simulink model "SIL_PIL_position_controller_model"  (R2023b)
settings: Solver=FixedStepAuto  StartTime=0.0  StopTime=10.0  RelTol=1e-3  EnableMultiTasking=on
undefined symbols (not defined in the file): DiscIntNeverNeededParam, K
settings Model: ExtModeTrigDuration=10  Creator=paoli  LastModifiedBy=paoli
settings OptimizationCC: EnhancedBackFolding=on  PassReuseOutputArgsAs=Individual arguments  ZeroExternalMemoryAtStartup=off  ZeroInternalMemoryAtStartup=off  MaxStackSize=64  OptimizeBlockOrder=speed  DifferentSizesBufferReuse=on  OptimizationCustomize=off  EfficientTunableParamExpr=on
settings DebuggingCC: ParameterTunabilityLossMsg=error
settings HardwareCC: ProdBitPerPointer=32  ProdBitPerSizeT=32  ProdBitPerPtrDiffT=32  ProdLargestAtomicInteger=Long  ProdLargestAtomicFloat=Double  ProdWordSize=32  ProdLongLongMode=on  ProdHWDeviceType=ARM Compatible->ARM Cortex
settings SFSimCC: MATLABDynamicMemAlloc=off
settings RTWCC: Description=Embedded Coder  SystemTargetFile=ert.tlc  HardwareBoard=STM32 Nucleo F401RE  TemplateMakefile=ert_default_tmf  Toolchain=GNU Tools for ARM Embedded Processors  PortableWordSizes=on
settings CodeAppCC: ForceParamTrailComments=on  IgnoreCustomStorageClasses=off  OperatorAnnotations=on  SimulinkDataObjDesc=on  SFDataObjDesc=on  InsertBlockDesc=on
settings ERTTargetCC: ExtModeTransport=3  ExtModeStaticAlloc=on  ExtModeStaticAllocSize=2000  ExtModeMexFile=ext_xcp  ExtModeIntrfLevel=Level2 - Open

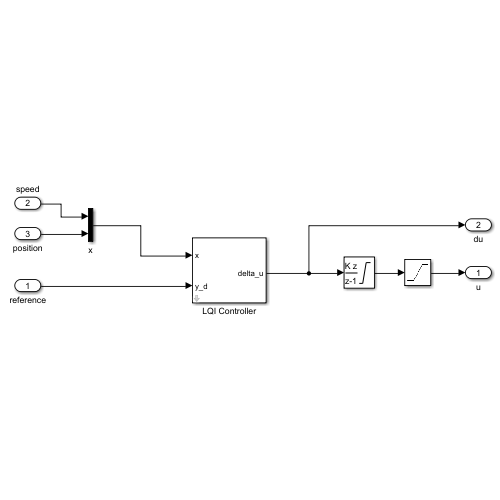
[thumbnail: Simulink's stored preview of the top-level diagram]
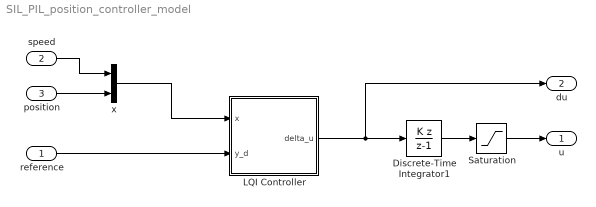
== system SIL_PIL_position_controller_model ==
  reference : Inport
  speed : Inport  Port=2
  position : Inport  Port=3
  Discrete-Time Integrator1 : DiscreteIntegrator  IntegratorMethod=Accumulation: Backward Euler  SampleTime=-1  LimitOutput=on  UpperSaturationLimit=12  LowerSaturationLimit=-12  ICPrevOutput=DiscIntNeverNeededParam  ICPrevScaledInput=DiscIntNeverNeededParam
  LQI Controller : Subsystem  mask{Ts=0.005}
  Saturation : Saturate  UpperLimit=12  LowerLimit=-12
  x : Mux  Inputs=2
  u : Outport
  du : Outport  Port=2
  wires:
  Discrete-Time Integrator1/1 -> Saturation/1
  LQI Controller/1(delta_u) -> du/1, Discrete-Time Integrator1/1
  Saturation/1 -> u/1
  reference/1 -> LQI Controller/2(y_d)
  speed/1 -> x/1
  position/1 -> x/2
  x/1 -> LQI Controller/1(x)

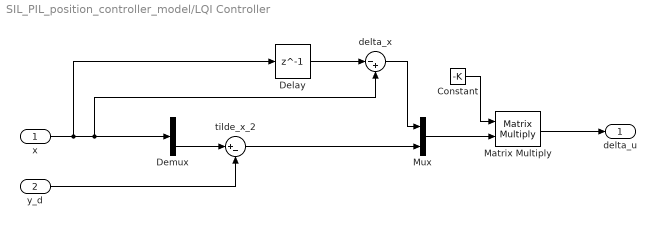
== system SIL_PIL_position_controller_model/LQI Controller ==
  x : Inport  SampleTime=Ts
  y_d : Inport  Port=2  SampleTime=Ts
  Constant : Constant  Value=-K  VectorParams1D=off
  Delay : Delay  DelayLength=1  InitialCondition=[0;0]  SampleTime=Ts
  Demux : Demux  Outputs=2
  Matrix Multiply : Product  Multiplication=Matrix(*)
  Mux : Mux  Inputs=2
  delta_x : Sum  Inputs=|-+
  tilde_x_2 : Sum  Inputs=|+-
  delta_u : Outport  SampleTime=Ts
  wires:
  x/1 -> Delay/1, delta_x/2, Demux/1
  Mux/1 -> Matrix Multiply/2
  Demux/2 -> tilde_x_2/1
  y_d/1 -> tilde_x_2/2
  Delay/1 -> delta_x/1
  tilde_x_2/1 -> Mux/2
  Matrix Multiply/1 -> delta_u/1
  Constant/1 -> Matrix Multiply/1
  delta_x/1 -> Mux/1
